simulink model "trajectorySimulation"  (R2015b)
settings: Solver=FixedStepAuto  StartTime=0.0  StopTime=15.13  FixedStep=1/60  RelTol=1e-3
libraries: aerolibfltsims x3, aerolibconvert2 x2, aerolibanimutils x1
settings Model: Creator=fidel  LastModifiedBy=fidel

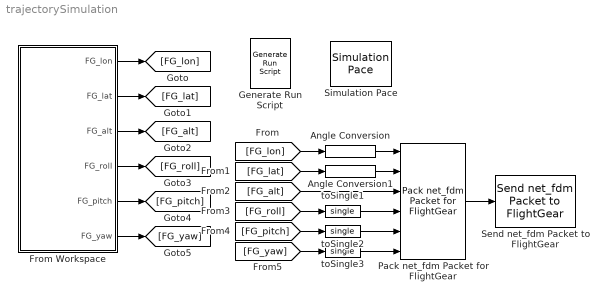
== system trajectorySimulation ==
  Angle Conversion : aerolibconvert2/Angle Conversion  IU=deg  OU=rad
  Angle Conversion1 : aerolibconvert2/Angle Conversion  IU=deg  OU=rad
  From Workspace : Subsystem
  Generate Run Script : aerolibfltsims/Generate Run Script  OutputFileName=optimFP_runFG.bat  FlightGearBaseDirectory=C:\Program Files\FlightGear 2016.4.4  GeometryModelName=ZivkoEdge540  DestinationPort=5502  OriginAddress=127.0.0.1  OriginPort=5505  LocalAddress=127.0.0.1  AirportId=KSFO  RunwayId=10L  InitialAltitude=7224  InitialHeading=113  OffsetDistance=4.72  OffsetAzimuth=0  GenerateFile=off  Architecture=Default  dataFlow=Send
  Pack net_fdm Packet for FlightGear : aerolibfltsims/Pack net_fdm Packet for FlightGear  FlightGearVersion=v3.4  ShowPositionAttitudeInputs=on  ShowVelocityAccelerationInputs=off  ShowControlSurfacePositionInputs=off  ShowEngineFuelInputs=off  ShowLandingGearInputs=off  ShowEnvironmentInputs=off  SampleTime=-1
  Send net_fdm Packet to FlightGear : aerolibfltsims/Send net_fdm Packet to FlightGear  DestinationIpAddress=127.0.0.1  DestinationPort=5502  LocalIpPort=-1  varLen=off  SampleTime=-1
  Simulation Pace : aerolibanimutils/Simulation Pace  SimulationPace=1  SleepMode=MATLAB Thread  OutputPaceError=off  SampleTime=-1
      settings: AttributesFormatString=%<SimulationPace> sec/sec
  toSingle1 : DataTypeConversion  OutDataTypeStr=single
  toSingle2 : DataTypeConversion  OutDataTypeStr=single
  toSingle3 : DataTypeConversion  OutDataTypeStr=single
  wires:
  Angle Conversion1/1 -> Pack net_fdm Packet for FlightGear/2
  Angle Conversion/1 -> Pack net_fdm Packet for FlightGear/1
  toSingle3/1 -> Pack net_fdm Packet for FlightGear/6
  toSingle2/1 -> Pack net_fdm Packet for FlightGear/5
  toSingle1/1 -> Pack net_fdm Packet for FlightGear/4
  Pack net_fdm Packet for FlightGear/1 -> Send net_fdm Packet to FlightGear/1
  From Workspace/1(FG_lon) -> [FG_lon]
  From Workspace/2(FG_lat) -> [FG_lat]
  From Workspace/3(FG_alt) -> [FG_alt]
  From Workspace/5(FG_pitch) -> [FG_pitch]
  [FG_yaw] -> toSingle3/1
  [FG_lon] -> Angle Conversion/1
  [FG_lat] -> Angle Conversion1/1
  [FG_alt] -> Pack net_fdm Packet for FlightGear/3
  [FG_roll] -> toSingle1/1
  [FG_pitch] -> toSingle2/1
  From Workspace/6(FG_yaw) -> [FG_yaw]
  From Workspace/4(FG_roll) -> [FG_roll]

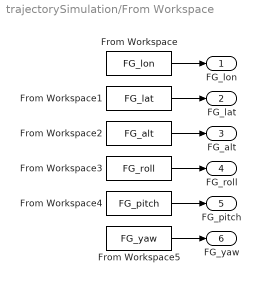
== system trajectorySimulation/From Workspace ==
  From Workspace : FromWorkspace  VariableName=FG_lon  SampleTime=0
  From Workspace1 : FromWorkspace  VariableName=FG_lat  SampleTime=0
  From Workspace2 : FromWorkspace  VariableName=FG_alt  SampleTime=0
  From Workspace3 : FromWorkspace  VariableName=FG_roll  SampleTime=0
  From Workspace4 : FromWorkspace  VariableName=FG_pitch  SampleTime=0
  From Workspace5 : FromWorkspace  VariableName=FG_yaw  SampleTime=0
  FG_lon : Outport
  FG_lat : Outport  Port=2
  FG_alt : Outport  Port=3
  FG_roll : Outport  Port=4
  FG_pitch : Outport  Port=5
  FG_yaw : Outport  Port=6
  wires:
  From Workspace4/1 -> FG_pitch/1
  From Workspace3/1 -> FG_roll/1
  From Workspace5/1 -> FG_yaw/1
  From Workspace/1 -> FG_lon/1
  From Workspace2/1 -> FG_alt/1
  From Workspace1/1 -> FG_lat/1
